simulink model "unifoil"  (R2018b)
settings: Solver=ode23s  StartTime=0.0  StopTime=T  RelTol=1e-3
undefined symbols (not defined in the file): addedInertia, addedMass, ARefElevator, ARefRudder, ARefWing, baseInertia, baseMass, basisParams, buoyFactor, density, flowSpeed, fuselageLength, initAzimuth, initElevation, initPathVar, initSpeed, initTwist, initTwistRate, maxIntAngle, maxLeadLength, p, radius, refGain1, refGain2, rudderAlphaMinusStall, rudderAlphaPlusStall, rudderCLCoeffs, rudderTable, tauRef, UNext, wingAlphaMinusStall, wingAlphaPlusStall, wingCDCoeffs, wingCLCoeffs, wingTable
libraries: vrlib x8, simulink x2
settings Model: SimulationMode=accelerator  Creator=mitch  LastModifiedBy=mitch

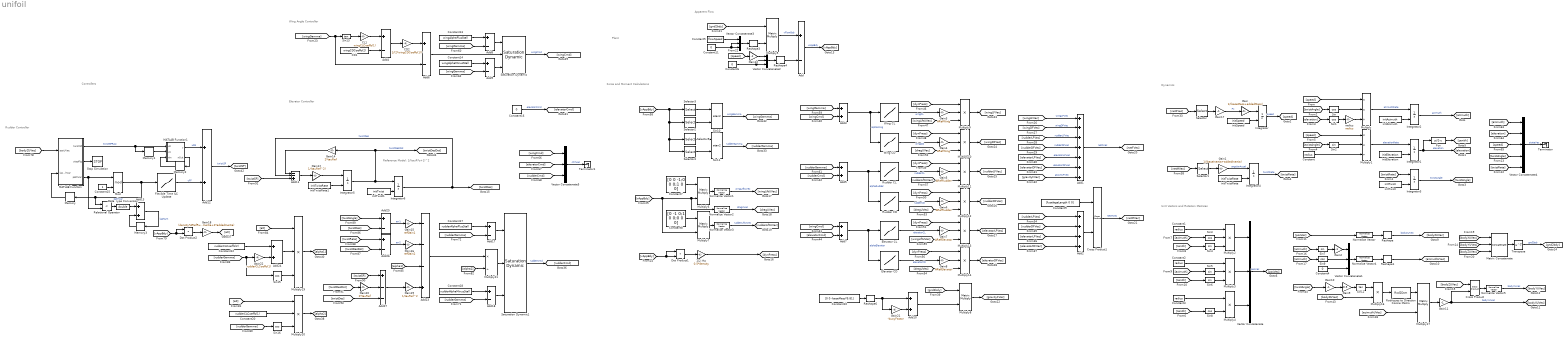
== system unifoil ==
  note: Plant
  note: Controllers
  note: Unit Vectors and Rotation Matrices
  note: Rudder Controller
  note: Dynamics
  note: Apparent Flow
  note: Elevator Controller
  note: Reference Model:
      | 1/(tauR*s+1)^2
  note: Force and Moment Calculations
  note: Wing Angle Controller
  1/2 rho : Gain  Gain=0.5*density
  Add{,4,6,8..9,17..18,25..26} (9 alike) : Sum  Inputs=+-
  Add1 : Sum  Inputs=+++++++
  Add{3,5,7,10,12..13,24} (7 alike) : Sum
  Add11 : Sum  Inputs=--+
  Add2 : Sum  Inputs=++++
  Add23 : Sum  Inputs=---+
  Add27 : Sum  Inputs=+--
  CD1 : Constant  Value=wingCDCoeffs(2)
  CD2 : Gain  Gain=1/(2*wingCDCoeffs(1))
  CL1 : Gain  Gain=wingCLCoeffs(1)
  Constant{,1..3} (4 alike) : Constant  Value=radius
  Constant10 : Constant  Value=[0 0 -baseMass*9.81]
  Constant{4,6,11,16} (4 alike) : Constant  Value=0
  Constant12 : Constant  Value=rudderCLCoeffs(2)
  Constant13 : Constant  Value=wingAlphaPlusStall
  Constant14 : Constant  Value=wingAlphaMinusStall
  Constant15 : Constant
  Constant17 : Constant  Value=rudderAlphaPlusStall
  Constant18 : Constant  Value=rudderAlphaMinusStall
  Constant20 : Constant  Value=rudderCLCoeffs(1)
  Constant5 : Constant  Value=flowSpeed
  Constant7 : Constant  Value=[0 0 -1;0 0 0;1 0 0]
  Constant8 : Constant  Value=[0 -1 0;1 0 0;0 0 0]
  Constant9 : Constant  Value=[fuselageLength 0 0]
  Cross Product : vrlib/Utilities/Cross Product
      settings: SourceProductBaseCode=VR
  Cross Product1 : vrlib/Utilities/Cross Product
      settings: SourceProductBaseCode=VR
  Data Type Conversion : DataTypeConversion  OutDataTypeStr=double
  Dot Product1 : DotProduct  InputSameDT=on  OutDataTypeStr=Inherit: Inherit via internal rule
  Dot Product2 : DotProduct  InputSameDT=on  OutDataTypeStr=Inherit: Inherit via internal rule
  Elevator CD : Lookup_n-D  NumberOfTableDimensions=1  BreakpointsForDimension1=rudderTable.alpha  Table=rudderTable.CD  InternalRulePriority=Speed  RndMeth=Simplest  InputSameDT=on
  Elevator CL : Lookup_n-D  NumberOfTableDimensions=1  BreakpointsForDimension1=rudderTable.alpha  Table=rudderTable.CL  InternalRulePriority=Speed  RndMeth=Simplest  InputSameDT=on
  Fcn : Fcn  Expr=pi/2-u
  Flexible Time ILC Update : Lookup_n-D  NumberOfTableDimensions=1  BreakpointsForDimension1=UNext.Time(:)  Table=UNext.Data(:)  ExtrapMethod=Clip  UseLastTableValue=on  InternalRulePriority=Speed  RndMeth=Simplest  InputSameDT=on
  Gain : Gain  Gain=1/(baseMass+addedMass)
  Gain1 : Gain  Gain=1/(baseInertia+addedInertia)
  Gain{2,10..12,17} (5 alike) : Gain  Gain=-1
  Gain13 : Gain  Gain=1/(tauRef^2)
  Gain14 : Gain  Gain=2*tauRef
  Gain15 : Gain  Gain=refGain1
      settings: AttributesFormatString=%<Gain>
  Gain16 : Gain  Gain=refGain2
      settings: AttributesFormatString=%<Gain>
  Gain18 : Gain  Gain=(density*ARefRudder*fuselageLength)/(2*baseInertia+2*addedInertia)
  Gain19 : Gain  Gain=1/tauRef^2
  Gain20 : Gain  Gain=2*tauRef
  Gain21 : Gain  Gain=-buoyFactor
      settings: AttributesFormatString=%<Gain>
  Gain22 : Gain  Gain=rudderCLCoeffs(1)
  Gain3 : Gain  Gain=ARefWing
      settings: AttributesFormatString=%<Gain>
  Gain4 : Gain  Gain=ARefWing
      settings: AttributesFormatString=%<Gain>
  Gain5 : Gain  Gain=ARefRudder
      settings: AttributesFormatString=%<Gain>
  Gain6 : Gain  Gain=ARefRudder
      settings: AttributesFormatString=%<Gain>
  Gain7 : Gain  Gain=ARefElevator
      settings: AttributesFormatString=%<Gain>
  Gain8 : Gain  Gain=ARefElevator
      settings: AttributesFormatString=%<Gain>
  Gain9 : Gain  Gain=0.5
  Integrator{,1..5} (6 alike) : Integrator  InitialConditionSource=external
  Integrator6 : Integrator  InitialConditionSource=external  InitialCondition=p.initTwist
  MATLAB Function : MATLAB Function  TreatAsAtomicUnit=on
  MATLAB Function1 : MATLAB Function  TreatAsAtomicUnit=on
  Matrix Concatenate : Concatenate  NumInputs=3  Mode=Multidimensional array  ConcatenateDimension=2
  Memory : Memory  InitialCondition=initPathVar
  Memory1 : Memory  InitialCondition=initTwist
  Memory2 : Memory
  Memory3 : Memory  InitialCondition=1
  Mod : Math  Operator=mod  SaturateOnIntegerOverflow=on
  Multiply : Product  Inputs=**/
  Multiply1 : Product  Inputs=**/
  Multiply{2..3,9..14,19..20} (10 alike) : Product  Inputs=3
  Multiply16 : Product
  Multiply{5..8,17} (5 alike) : Product  Multiplication=Matrix(*)
  Multiply21 : Product  Inputs=*/
  Multiply4 : Product
  Normalize Vector{,1..5} (6 alike) : vrlib/Utilities/Normalize Vector  maxzero=0
      settings: SourceProductName=Simulink 3D Animation  SourceProductBaseCode=VR
  Relational Operator : RelationalOperator  Operator=<  OutDataTypeStr=boolean  RndMeth=Simplest
  Reshape{,1,3..4,6} (5 alike) : Reshape  OutputDimensionality=Column vector (2-D)
  Rodrigues to Direction Cosine Matrix : Rod2Dcm
  Rudder CD : Lookup_n-D  NumberOfTableDimensions=1  BreakpointsForDimension1=rudderTable.alpha  Table=rudderTable.CD  InternalRulePriority=Speed  RndMeth=Simplest  InputSameDT=on
  Rudder CL : Lookup_n-D  NumberOfTableDimensions=1  BreakpointsForDimension1=rudderTable.alpha  Table=rudderTable.CL  InternalRulePriority=Speed  RndMeth=Simplest  InputSameDT=on
  Saturation Dynamic : simulink/Discontinuities/Saturation Dynamic  OutMin=[]  OutMax=[]  OutDataTypeStr=Inherit: Same as second input  OutDataType=fixdt(1, 16)  OutScaling=2^-10  DoSatur=off
  Saturation Dynamic1 : simulink/Discontinuities/Saturation Dynamic  OutMin=[]  OutMax=[]  OutDataTypeStr=Inherit: Same as second input  OutDataType=fixdt(1, 16)  OutScaling=2^-10  DoSatur=off
  Selector : Selector  InputPortWidth=3  IndexOptions=Index vector (dialog)  Indices=1  OutputSizes=1
  Selector1 : Selector  InputPortWidth=3  IndexOptions=Index vector (dialog)  Indices=3  OutputSizes=1
  Selector2 : Selector  InputPortWidth=3  IndexOptions=Index vector (dialog)  Indices=1  OutputSizes=1
  Selector3 : Selector  InputPortWidth=3  IndexOptions=Index vector (dialog)  Indices=3  OutputSizes=1
  Selector4 : Selector  InputPortWidth=3  IndexOptions=Index vector (dialog)  Indices=1  OutputSizes=1
  Selector5 : Selector  InputPortWidth=3  IndexOptions=Index vector (dialog)  Indices=2  OutputSizes=1
  Sin{,1,3,8..9,15..16} (7 alike) : Trigonometry  Operator=cos
  Sin10 : Trigonometry  Operator=atan2
  Sin11 : Trigonometry  Operator=atan2
  Sin12 : Trigonometry  Operator=tan
  Sin13 : Trigonometry  Operator=tan
  Sin{2,4..7} (5 alike) : Trigonometry
  Stop Simulation : Stop
  Terminator : Terminator
  Terminator1 : Terminator
  Transpose : Math  Operator=transpose  SaturateOnIntegerOverflow=on
  Vector Concatenate : Concatenate  NumInputs=3  Mode=Multidimensional array
  Vector Concatenate{1..3,5} (4 alike) : Concatenate  NumInputs=3
  Vector Concatenate4 : Concatenate  NumInputs=5  Mode=Multidimensional array
  Wing CD : Lookup_n-D  NumberOfTableDimensions=1  BreakpointsForDimension1=wingTable.alpha  Table=wingTable.CD  InternalRulePriority=Speed  RndMeth=Simplest  InputSameDT=on
  Wing CL : Lookup_n-D  NumberOfTableDimensions=1  BreakpointsForDimension1=wingTable.alpha  Table=wingTable.CL  InternalRulePriority=Speed  RndMeth=Simplest  InputSameDT=on
  initAzimuth : Constant  Value=initAzimuth
  initElevation : Constant  Value=initElevation
  initSpeed : Constant  Value=initSpeed
  initTwist : Constant  Value=initTwist
  initTwist1 : Constant  Value=initTwist
  initTwistRate : Constant  Value=initTwistRate
  initTwistRate1 : Constant  Value=initTwistRate
  radius : Gain  Gain=radius
  wires:
  initSpeed/1 -> Integrator/2
  initElevation/1 -> Integrator1/2
  initAzimuth/1 -> Integrator2/2
  initTwist/1 -> Integrator3/2
  initTwistRate/1 -> Integrator4/2
  Integrator4/1 -> [twistRate]  "twistRate"
  Integrator2/1 -> [azimuth]  "azimuth"
  Integrator/1 -> [speed]  "speed"
  Multiply/1 -> Integrator2/1  "azimuthRate"
  [speed] -> Multiply/1
  Integrator3/1 -> [twistAngle]  "twistAngle"
  [twistRate] -> Integrator3/1
  Sin/1 -> Multiply/2
  [twistAngle] -> Sin/1
  radius/1 -> Multiply/3
  Sin1/1 -> radius/1
  [elevation] -> Sin1/1
  Multiply1/1 -> Integrator1/1  "elevationRate"
  [twistAngle] -> Sin2/1
  Sin2/1 -> Multiply1/2
  [speed] -> Multiply1/1
  Constant/1 -> Multiply1/3
  Integrator1/1 -> Fcn/1, [elevation]  "elevation"
  Fcn/1 -> [zenith]
  Constant1/1 -> Multiply2/1
  [azimuth] -> Sin3/1
  Sin3/1 -> Multiply2/2
  Sin4/1 -> Multiply2/3
  [zenith] -> Sin4/1
  Multiply2/1 -> Vector Concatenate/1
  Multiply3/1 -> Vector Concatenate/2
  [zenith] -> Sin6/1
  Sin6/1 -> Multiply3/3
  Sin5/1 -> Multiply3/2
  [azimuth] -> Sin5/1
  Constant2/1 -> Multiply3/1
  Constant3/1 -> Multiply4/1
  [zenith] -> Sin8/1
  Sin8/1 -> Multiply4/2
  Multiply4/1 -> Vector Concatenate/3
  Gain/1 -> Integrator/1
  Gain1/1 -> Integrator4/1  "angularAccel"
  Normalize Vector/1 -> Reshape/1
  Reshape/1 -> [bodyZUVec]  "bodyZUVec"
  Vector Concatenate1/1 -> Normalize Vector4/1
  Reshape1/1 -> [azimuthUVec]
  Gain2/1 -> Vector Concatenate1/1
  Sin7/1 -> Gain2/1
  Sin9/1 -> Vector Concatenate1/2
  Constant4/1 -> Vector Concatenate1/3
  [azimuth] -> Sin7/1
  [azimuth] -> Sin9/1
  Reshape3/1 -> Multiply5/2
  [gnd2bdy] -> Multiply5/1
  Multiply5/1 -> Add/1  "vFlowBdy"
  [speed] -> Gain12/1
  Constant6/1 -> Vector Concatenate2/2, Vector Concatenate2/3
  Vector Concatenate2/1 -> Reshape4/1
  Reshape4/1 -> Add/2
  Add/1 -> [vAppBdy]  "vAppBdy"
  [vAppBdy] -> Dot Product1/1, Dot Product1/2
  Dot Product1/1 -> 1/2 rho/1
  Constant7/1 -> Multiply6/1
  Multiply6/1 -> Normalize Vector1/1
  [vAppBdy] -> Multiply7/2, Normalize Vector2/1, Multiply6/2
  Constant8/1 -> Multiply7/1
  Multiply7/1 -> Normalize Vector3/1
  Normalize Vector1/1 -> [wingLiftUVec]  "wingLiftUVec"
  Normalize Vector2/1 -> [dragUVec]  "dragUVec"
  Normalize Vector3/1 -> [rudderLiftUVec]  "rudderLiftUVec"
  [rudderDFVec] -> Add1/4  "rudderDFVec"
  [rudderLFVec] -> Add1/3  "rudderLFVec"
  [wingDFVec] -> Add1/2  "wingDFVec"
  [wingLFVec] -> Add1/1  "wingLFVec"
  [elevatorLFVec] -> Add1/5  "elevatorLFVec"
  [elevatorDFVec] -> Add1/6  "elevatorDFVec"
  Add1/1 -> [netFVec]  "netFVec"
  [gravityFVec] -> Add1/7  "gravityFVec"
  [netFVec] -> Selector/1
  Constant9/1 -> Cross Product1/1
  Add2/1 -> Cross Product1/2
  [elevatorDFVec] -> Add2/4
  [elevatorLFVec] -> Add2/3
  [rudderLFVec] -> Add2/1
  [rudderDFVec] -> Add2/2
  [netMVec] -> Selector1/1
  Selector1/1 -> Gain1/1
  Cross Product1/1 -> [netMVec]  "netMVec"
  Multiply8/1 -> [gravityFVec]
  [gnd2bdy] -> Multiply8/1
  Reshape6/1 -> Add10/1, Gain21/1
  Constant10/1 -> Reshape6/1
  [wingCmd] -> Add3/2
  Add3/1 -> Wing CD/1, Wing CL/1  "alphaWing"
  [rudderCmd] -> Add5/2
  Add5/1 -> Rudder CD/1, Rudder CL/1  "alphaRudder"
  Add7/1 -> Elevator CL/1, Elevator CD/1  "alphaElevator"
  [elevatorCmd] -> Add7/2
  1/2 rho/1 -> [dynPress]
  Wing CL/1 -> Gain3/1  "wingCL"
  [dynPress] -> Multiply9/1
  [wingLiftUVec] -> Multiply9/3
  [dynPress] -> Multiply10/1
  Wing CD/1 -> Gain4/1  "wingCD"
  [dynPress] -> Multiply11/1
  Rudder CL/1 -> Gain5/1  "rudderCL"
  [dynPress] -> Multiply12/1
  Rudder CD/1 -> Gain6/1  "rudderCD"
  [dynPress] -> Multiply13/1
  Elevator CL/1 -> Gain7/1  "elevatorCL"
  Elevator CD/1 -> Gain8/1  "elevatorCD"
  [dragUVec] -> Multiply10/3
  [dragUVec] -> Multiply12/3
  [dragUVec] -> Multiply14/3
  [wingLiftUVec] -> Multiply13/3
  [dynPress] -> Multiply14/1
  [rudderLiftUVec] -> Multiply11/3
  Multiply9/1 -> [wingLFVec]
  Multiply10/1 -> [wingDFVec]
  Multiply11/1 -> [rudderLFVec]
  Multiply12/1 -> [rudderDFVec]
  Selector2/1 -> Sin10/2
  Selector3/1 -> Sin10/1
  [wingGamma] -> Add3/1
  Sin10/1 -> [wingGamma]  "wingGamma"
  Sin11/1 -> [rudderGamma]  "rudderGamma"
  [vAppBdy] -> Selector5/1, Selector4/1, Selector2/1, Selector3/1
  Selector5/1 -> Sin11/1
  Selector4/1 -> Sin11/2
  [rudderGamma] -> Add5/1
  [wingCmd] -> Add7/1
  Vector Concatenate3/1 -> Reshape3/1
  Constant5/1 -> Vector Concatenate3/1
  Constant11/1 -> Vector Concatenate3/2, Vector Concatenate3/3
  Gain3/1 -> Multiply9/2
  Gain4/1 -> Multiply10/2
  Gain5/1 -> Multiply11/2
  Gain6/1 -> Multiply12/2
  Gain7/1 -> Multiply13/2
  Gain8/1 -> Multiply14/2
  Matrix Concatenate/1 -> Transpose/1
  Transpose/1 -> [gnd2bdy]  "gnd2bdy"
  [bodyZUVec] -> Matrix Concatenate/3
  [bodyZUVec] -> Multiply16/2
  [twistAngle] -> Gain10/1
  Gain9/1 -> Sin12/1
  Sin12/1 -> Multiply16/1
  Multiply16/1 -> Rodrigues to Direction Cosine Matrix/1
  Rodrigues to Direction Cosine Matrix/1 -> Multiply17/1
  Multiply17/1 -> Gain11/1
  [azimuthUVec] -> Multiply17/2
  [bodyYUVec] -> Matrix Concatenate/2
  [bodyZUVec] -> Cross Product/1
  Cross Product/1 -> Normalize Vector5/1
  [bodyXUVec] -> Matrix Concatenate/1
  Gain11/1 -> Cross Product/2, [bodyXUVec]  "bodyXUVec"
  Gain10/1 -> Gain9/1
  Normalize Vector4/1 -> Reshape1/1
  Normalize Vector5/1 -> [bodyYUVec]  "bodyYUVec"
  Gain12/1 -> Vector Concatenate2/1
  [wingGamma] -> Add6/2, Sin13/1
  Sin13/1 -> CL1/1
  CL1/1 -> Add4/1
  CD1/1 -> Add4/2
  Add4/1 -> CD2/1
  CD2/1 -> Add6/1
  Saturation Dynamic/1 -> [wingCmd]  "wingCmd"
  Selector/1 -> Gain17/1
  Add6/1 -> Saturation Dynamic/2
  Add8/1 -> Saturation Dynamic/1
  Add9/1 -> Saturation Dynamic/3
  [wingGamma] -> Add8/2
  [wingGamma] -> Add9/2
  Constant13/1 -> Add8/1
  Constant14/1 -> Add9/1
  Add10/1 -> Multiply8/2
  Gain21/1 -> Add10/2
  Gain14/1 -> Add11/1
  Integrator5/1 -> Integrator6/1, [twistDesDot], Gain14/1  "twistDesDot"
  Integrator6/1 -> Add11/2, [twistDes]  "twistDes"
  Add11/1 -> Gain13/1
  Gain13/1 -> Integrator5/1
  Constant18/1 -> Add18/1
  Constant17/1 -> Add17/1
  [rudderGamma] -> Add17/2
  Add18/1 -> Saturation Dynamic1/3
  Add17/1 -> Saturation Dynamic1/1
  [rudderGamma] -> Add18/2
  Saturation Dynamic1/1 -> [rudderCmd]  "rudderCmd"
  initTwistRate1/1 -> Integrator5/2
  initTwist1/1 -> Integrator6/2
  Multiply13/1 -> [elevatorLFVec]
  Multiply14/1 -> [elevatorDFVec]
  Constant16/1 -> [elevatorCmd]  "elevatorCmd"
  [bodyZUVec] -> MATLAB Function/1(posUVec)
  MATLAB Function/3(pathVar) -> Relational Operator/2, Mod/1
  Memory/1 -> MATLAB Function/2(lastPathVar)
  Multiply21/1 -> Saturation Dynamic1/2
  [vAppBdy] -> Dot Product2/1, Dot Product2/2
  Dot Product2/1 -> Gain18/1
  Gain18/1 -> [a0]
  [a0] -> Multiply19/1
  Add24/1 -> Multiply19/2
  [rudderGamma] -> Sin15/1, Gain22/1
  Gain22/1 -> Add24/2
  Constant12/1 -> Add24/1
  Sin15/1 -> Multiply19/3
  Multiply19/1 -> [alpha1]
  Multiply20/1 -> [alpha2]
  Sin16/1 -> Multiply20/3
  [a0] -> Multiply20/1
  [rudderGamma] -> Sin16/1
  Constant20/1 -> Multiply20/2
  [alpha2] -> Multiply21/2
  Add23/1 -> Multiply21/1
  [alpha1] -> Add23/3
  [twistRate] -> Add26/1
  Add25/1 -> Gain15/1  "err1"
  Add26/1 -> Gain16/1  "err2"
  [twistDesDot] -> Add26/2
  [twistDes] -> Add25/2
  [twistAngle] -> Add25/1
  Gain19/1 -> Add23/4
  Add27/1 -> Gain19/1
  [twistSP] -> Add27/1
  Gain20/1 -> Add27/2
  [twistDesDot] -> Gain20/1
  [twistSP] -> Add11/3
  [twistDes] -> Add27/3
  Vector Concatenate/1 -> [posVec]  "posVec"
  [posVec] -> Normalize Vector/1
  Vector Concatenate4/1 -> Terminator/1  "stateVec"
  [twistRate] -> Vector Concatenate4/5
  [twistAngle] -> Vector Concatenate4/4
  [azimuth] -> Vector Concatenate4/1
  [elevation] -> Vector Concatenate4/2
  [speed] -> Vector Concatenate4/3
  Vector Concatenate5/1 -> Terminator1/1  "ctrlVec"
  [rudderCmd] -> Vector Concatenate5/3
  [elevatorCmd] -> Vector Concatenate5/2
  [wingCmd] -> Vector Concatenate5/1
  Gain15/1 -> Add23/1
  Gain16/1 -> Add23/2
  MATLAB Function/1(twistSP) -> Memory1/1, MATLAB Function1/1(u0)  "twistSPRaw"
  Memory1/1 -> MATLAB Function1/2(u1)
  MATLAB Function1/2(nOut) -> Memory2/1
  Memory2/1 -> MATLAB Function1/3(nIn)
  MATLAB Function/2(stopFlg) -> Stop Simulation/1
  Add12/1 -> [twistSP]  "twistSP"
  Flexible Time ILC Update/1 -> Add12/2  "uFF"
  MATLAB Function1/1(y) -> Add12/1  "uFB"
  Mod/1 -> Relational Operator/1, Memory/1, Flexible Time ILC Update/1  "pathVar"
  Constant15/1 -> Mod/2
  Relational Operator/1 -> Data Type Conversion/1
  Data Type Conversion/1 -> Add13/1
  Memory3/1 -> Add13/2
  Add13/1 -> Memory3/1  "lapNum"
  Gain17/1 -> Gain/1  "Fx"

== matlab function unifoil/MATLAB Function1 ==
  data: u0 input; y output; u1 input; nIn input; nOut output
function [y,nOut] = fcn(u0,u1,nIn)
% This function basically does what the simulink unwrap block should do,
% but that block seemed to be resampling to a slower time step, so I wrote
% this.
nOut = nIn;
% If there's a big negative jump
if u1-u0 > pi
    nOut = nIn+1;
end
% If there's a big positive jump
if u0-u1 > pi
    nOut = nIn-1;
end
% Add the appropriate number of 2pi offsets
y = u0 + 2*pi*nOut;

== matlab function unifoil/MATLAB Function ==
  data: posUVec input; twistSP output; stopFlg output; pathVar output; basisParams parameter; lastPathVar input; maxIntAngle parameter; maxLeadLength parameter
function [twistSP,stopFlg,pathVar] = fcn(posUVec,basisParams, ...
    lastPathVar, maxIntAngle, maxLeadLength)

% Start 1D maximization (via Golden Section) from here
gr = ((sqrt(5)+1)/2);
s1 = lastPathVar - 0.1;
s4 = lastPathVar + 0.1;
[J1,p1] = perfIndx(s1,basisParams,posUVec);
[J4,p4] = perfIndx(s4,basisParams,posUVec);

s3 = s1 + (s4-s1)/gr;
s2 = s4 - (s4-s1)/gr;
[J3,p3] = perfIndx(s3,basisParams,posUVec);
[J2,p2] = perfIndx(s2,basisParams,posUVec);
% plot([s1 s2 s3 s4],[J1 J2 J3 J4])
for ii = 1:100 % Max 100 iterations
    if J2<J3
        % Overwrite 1 with 2
        s1 = s2;
        J1 = J2;
        p1 = p2;
        % Overwrite 2 with 3
        s2 = s3;
        J2 = J3;
        p2 = p3;
        % Recalculate 3
        s3 = s1 + (s4-s1)/gr;
        [J3,p3] = perfIndx(s3,basisParams,posUVec);
    else
        % Overwrite 4 with 3
        s4 = s3;
        J4 = J3;
        p4 = p3;
        % Overwrite 3 with 2
        s3 = s2;
        J3 = J2;
        p3 = p2;
        % Recalculate 2
        s2 = s4 - (s4-s1)/gr;
        [J2,p2] = perfIndx(s2,basisParams,posUVec);
    end
    % If length of path spanned by search region is too small
    if sqrt(sum((p4-p1).^2))<1e-4 
        break
    end
end
pathVar = (s4+s1)/2;
stopFlg = pathVar>mod(pathVar,1);
% pathVar = mod(pathVar,1);
intAng  = acos((J4+J1)/2);
% Weight varies 0->1 as distance from path increases
% wght = 1 means head straight at path
wght            = max([min([intAng/maxIntAngle,1]),0]);
% Calculate lead length
% leadLength      = maxLeadLength*(1-wght);
leadLength      = maxLeadLength;
targetPT        = lemOfGerono(pathVar+leadLength,basisParams);
targetPTUVec    = targetPT./sqrt(sum(targetPT.^2));
twistSP         = heading(posUVec,targetPTUVec);
end


function [J,pathVec] = perfIndx(s,basisParams,posUVec)
pathVec = lemOfGerono(s,basisParams);
J = dot(pathVec./sqrt(sum(pathVec.^2)),posUVec);
end
